simulink model "genericjosephtest"  (Simulink 10.3)
settings: Solver=ode45  StartTime=0.0  StopTime=inf  RelTol=1e-3  EnableMultiTasking=on
values from neighbouring files (symbols this model uses):
  ku = (Lr*m)/(Cyf*(Lf+Lr)) - (Lf*m)/(Cyr*(Lf+Lr))    (= -0.00270204285714)    [makePlants.m]
  Lf = 0.918    [makeBikeModel.m]    (also in makePlants.m)
  Lr = 0.612    [makeBikeModel.m]    (also in makePlants.m)
undefined symbols (not defined in the file or in its folder): Gains
libraries: CarMaker4SL x24, slctrlblks x2, pid_lib x2, simulink x1
(part 2 of 3)

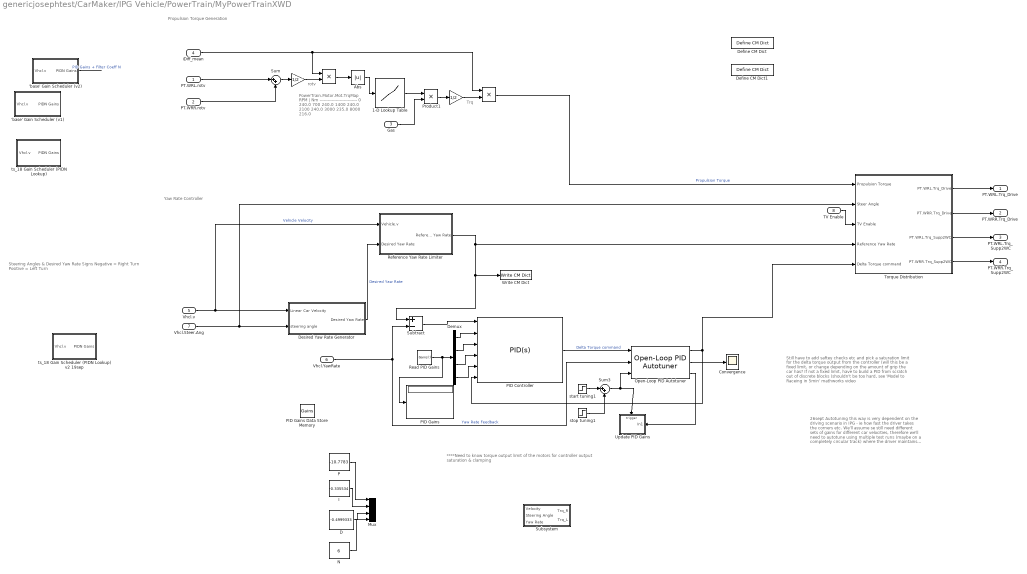
== system genericjosephtest/CarMaker/IPG Vehicle/PowerTrain/MyPowerTrainXWD ==
  note: 26sept
      |
      | Autotuning this way is very dependent on the driving scenario in IPG - ie how fast the driver takes the corners etc. We'll assume se still need different sets of gains for different car velocities, therefore we'll need to autotune using multiple test runs (maybe on a completely circular track) where the driver maintains different cruising speeds each time. Also, need to be mindful of when the start-stop time for the autotuning to ensure the controller is tuned for the correct scenario (ie mid-turn and a relatively constant speed rather than accelerating from a standstill).
      |
      | **also investigate some weird spikes and behaviour of the reference/desired yaw rate generators
  note: Propulsion Torque Generation
  note: ****Need to know torque output limit of the motors for controller output saturation & clamping
  note: Still have to add saftey checks etc and pick a saturation limit for the delta torque output from the controller (will this be a fixed limit, or change depending on the amount of grip the car has? If not a fixed limit, have to build a PID from scratch out of discrete blocks (shouldn't be too hard, see 'Model to Raceing in 5min' mathworks video
  note: Steering Angles & Desired Yaw Rate Signs
      |
      | Negative = Right Turn
      | Positive = Left Turn
  note: rotv
  note: Trq
  note: PowerTrain.Motor.Mot.TrqMap
      |
      |     RPM |  Nm
      | ----------------------------
      |     0         240.0
      |     700     240.0
      |     1400   240.0
      |     2100   240.0
      |     3000   235.0
      |     8000   216.0
  note: Yaw Rate Controller
  PT.WRL.rotv : Inport
  PT.WRR.rotv : Inport  Port=2
  Gas : Inport  Port=3
  iDiff_mean : Inport  Port=4
  Vhcl.v : Inport  Port=5
  Vhcl.YawRate : Inport  Port=6
  Vhcl.Steer.Ang : Inport  Port=7
  TV Enable : Inport  Port=8
  " " : Gain  Gain=1/2
  "  " : Gain  Gain=1/2
  "   " : Product
  "    " : Product
  'base' Gain Scheduler (v1) : Subsystem
  'base' Gain Scheduler (v2) : Subsystem
  1-D Lookup Table : Lookup_n-D  NumberOfTableDimensions=1  BreakpointsForDimension1=[0,700,1400,2100,3000,8000]  Table=[240,240,240,240,235,216]  InternalRulePriority=Speed  RndMeth=Simplest  InputSameDT=on
  Abs : Abs
  Convergence : Scope
  D : Constant  Value=-0.4999333
  Define CM Dict : CarMaker4SL/Define CM Dict  xname=RefYawRate  xunit=rad/s  xmono=off  xtype=Double4  xdvaplace=None  xnstates=0  xfirststate=0  xinitial=0
  Define CM Dict1 : CarMaker4SL/Define CM Dict  xname=DesYawRate  xunit=rad/s  xmono=off  xtype=Double4  xdvaplace=None  xnstates=0  xfirststate=0  xinitial=0
  Demux : Demux
  Desired Yaw Rate Generator : Subsystem
  I : Constant  Value=-0.335534
  Mux : Mux
  N : Constant  Value=6
  Open-Loop PID Autotuner : slctrlblks/Open-Loop PID Autotuner  PIDType=PIDF  PIDForm=Parallel  TimeDomain=discrete-time  DiscreteTs=0.1  IntegratorFormula=Forward Euler  FilterFormula=Forward Euler  ContinuousTs=0.02  Bandwidth=2  UseExternalWC=off  TargetPM=60  UseExternalPM=off  UseExternalAchievedPM=off  AmpSine=0.1  UseExternalAmpSine=off  EstimateDCGain=on  AmpStep=0.1  UseExternalAmpStep=off  UseExternalFRD=off  UseExternalU0=off  UseExternalDCGain=off  NotDeployTuningModule=off  UsePLCCoder=off  BlockDataType=double  UseConnectedPID=on  blockpath=[]  tunedP=0  tunedI=0  tunedD=0  tunedN=100  tunedPM=0  EstimationWindowSize=4
      settings: SourceProductBaseCode=SD
  P : Constant  Value=-10.7783
  "PID Controller " : pid_lib/PID Controller  Controller=PID  Form=Parallel  TimeDomain=Continuous-time  UseExternalTs=off  SampleTime=-1  IntegratorMethod=Forward Euler  FilterMethod=Forward Euler  ControllerParametersSource=external  P=140  I=2312  D=0.85  UseFilter=on  N=47  TunerSelectOption=Transfer Function Based (PID Tuner App)  InitialConditionSource=internal  InitialConditionForIntegrator=0  InitialConditionForFilter=0  DifferentiatorICPrevScaledInput=0  ExternalReset=none  TrackingMode=on  Kt=1  LimitOutput=off  SatLimitsSource=internal  UpperSaturationLimit=240  LowerSaturationLimit=0  LinearizeAsGain=off  AntiWindupMode=clamping  Kb=1  POutMin=[]  POutMax=[]  IOutMin=[]  IOutMax=[]  DOutMin=[]  DOutMax=[]  NOutMin=[]  NOutMax=[]  SumOutMin=[]  SumOutMax=[]  SaturationOutMin=[]  SaturationOutMax=[]  PParamMin=[]  PParamMax=[]  IParamMin=[]  IParamMax=[]  DParamMin=[]  DParamMax=[]  NParamMin=[]  NParamMax=[]  KbParamMin=[]  KbParamMax=[]  KtParamMin=[]  KtParamMax=[]  KbOutMin=[]  KbOutMax=[]  KtOutMin=[]  KtOutMax=[]  IntegratorOutMin=[]  IntegratorOutMax=[]  FilterOutMin=[]  FilterOutMax=[]  SumI1OutMin=[]  SumI1OutMax=[]  SumI2OutMin=[]  SumI2OutMax=[]  SumI3OutMin=[]  SumI3OutMax=[]  SumI4OutMin=[]  SumI4OutMax=[]  SumDOutMin=[]  SumDOutMax=[]  DifferentiatorOutMin=[]  DifferentiatorOutMax=[]  FilterDiffOutCoefMin=[]  FilterDiffOutCoefMax=[]  ReciprocalOutMin=[]  ReciprocalOutMax=[]  SumDenOutMin=[]  SumDenOutMax=[]  SumNumOutMin=[]  SumNumOutMax=[]  DivideOutMin=[]  DivideOutMax=[]  UdiffTsProdOutMin=[]  UdiffTsProdOutMax=[]  NTsProdOutMin=[]  NTsProdOutMax=[]  UintegralTsProdOutMin=[]  UintegralTsProdOutMax=[]  UngainTsProdOutMin=[]  UngainTsProdOutMax=[]  IntegratorContinuousStateAttributes=''  IntegratorStateMustResolveToSignalObject=off  IntegratorRTWStateStorageClass=Auto  FilterContinuousStateAttributes=''  FilterStateMustResolveToSignalObject=off  FilterRTWStateStorageClass=Auto  ParallelPVariant=ExternalParameters  IdealPVariant=Disabled  IVariant=ExternalParameters  DVariant=ExternalParameters  IntegratorVariant=Continuous  SatVariant=Disabled  AWVariant=Passthrough  PCopyVariant=Disabled  TRVariant=Enabled  FdbkBlocksVariant=Forward  IdealPFdbkVariant=Disabled  SatFdbkVariant=Disabled  DerivativeFilterVariant=ContFilter  NVariant=ExternalParameters  NCopyVariant=Disabled  FilterICVariant=InternalICsFilter  IntegratorICVariant=InternalICs  ExternalResetVariant=Disabled  TRSumVariant=TrackingMode  SumFdbkVariant=Disabled  SumVariant=Sum_PID  TsampFilterVariant=InternalTs  TsampNgainVariant=Passthrough  TsampIntegralVariant=Passthrough  ExternalSaturationOutDataTypeStr=Inherit: Same as second input
  PID Gains : Display
      settings: Decimation=5
  PID Gains Data Store Memory : DataStoreMemory  DataStoreName=Gains  InitialValue=[120 120 120 120]  ShowAdditionalParam=off
  Product1 : Product  RndMeth=Zero
  Read PID Gains : DataStoreRead  DataStoreName=Gains  DataStoreElements=Gains(:)  IndexOptions=Index vector (dialog)  Indices=1  OutputSizes=1
  Reference Yaw Rate Limiter : Subsystem
  Subsystem : Subsystem
  Subtract : Sum  Inputs=+-
  Sum : Sum  Inputs=|++
  Sum3 : Sum  Inputs=|++
  Torque Distribution : Subsystem
  Update PID Gains : Subsystem
  Write CM Dict : CarMaker4SL/Write CM Dict  xname=RefYawRate  xsync=off
  start tuning1 : Step  Time=10  SampleTime=0
  stop tuning1 : Step  Time=28  After=-1  SampleTime=0
  ts_18 Gain Scheduler (PIDN Lookup) : Subsystem
  ts_18 Gain Scheduler (PIDN Lookup) v2 19sep : Subsystem
  PT.WRL.Trq_Drive : Outport  VectorParamsAs1DForOutWhenUnconnected=off
  PT.WRR.Trq_Drive : Outport  Port=2  VectorParamsAs1DForOutWhenUnconnected=off
  PT.WRL.Trq_Supp2WC : Outport  Port=3  VectorParamsAs1DForOutWhenUnconnected=off
  PT.WRR.Trq_Supp2WC : Outport  Port=4  VectorParamsAs1DForOutWhenUnconnected=off
  wires:
  "  "/1 -> "   "/2
  Product1/1 -> "  "/1
  Gas/1 -> Product1/2
  1-D Lookup Table/1 -> Product1/1
  "    "/1 -> Abs/1
  iDiff_mean/1 -> "   "/1, "    "/1
  " "/1 -> "    "/2
  Sum/1 -> " "/1
  PT.WRR.rotv/1 -> Sum/2
  PT.WRL.rotv/1 -> Sum/1
  Abs/1 -> 1-D Lookup Table/1
  Vhcl.v/1 -> Desired Yaw Rate Generator/1(Linear Car Velocity), Reference Yaw Rate Limiter/1(Vehicle.v)  "Vehicle Velocity"
  Vhcl.Steer.Ang/1 -> Torque Distribution/2(Steer Angle), Desired Yaw Rate Generator/2(steering angle)
  Desired Yaw Rate Generator/1(Desired Yaw Rate) -> Reference Yaw Rate Limiter/2(Desired Yaw Rate)  "Desired Yaw Rate"
  Vhcl.YawRate/1 -> Open-Loop PID Autotuner/2, Subtract/2  "Yaw Rate Feedback"
  "   "/1 -> Torque Distribution/1(Propulsion Torque)  "Propulsion Torque"
  TV Enable/1 -> Torque Distribution/3(TV Enable)
  Torque Distribution/1(PT.WRL.Trq_Drive) -> PT.WRL.Trq_Drive/1
  Torque Distribution/2(PT.WRR.Trq_Drive) -> PT.WRR.Trq_Drive/1
  Torque Distribution/3(PT.WRL.Trq_Supp2WC) -> PT.WRL.Trq_Supp2WC/1
  Torque Distribution/4(PT.WRR.Trq_Supp2WC) -> PT.WRR.Trq_Supp2WC/1
  Reference Yaw Rate Limiter/1(Reference Yaw Rate) -> Write CM Dict/1, Subtract/1, Torque Distribution/4(Reference Yaw Rate)
  Demux/1 -> "PID Controller "/2
  Demux/2 -> "PID Controller "/3
  Demux/3 -> "PID Controller "/4
  Demux/4 -> "PID Controller "/5
  Subtract/1 -> "PID Controller "/1
  'base' Gain Scheduler (v2)/1(PIDN Gains) -> ?  "PID Gains + Filter Coeff N"
  Read PID Gains/1 -> Demux/1, PID Gains/1
  stop tuning1/1 -> Sum3/2
  start tuning1/1 -> Sum3/1
  Sum3/1 -> Update PID Gains/Trigger, Open-Loop PID Autotuner/3
  Open-Loop PID Autotuner/3 -> Update PID Gains/1(In1)
  Open-Loop PID Autotuner/2 -> Convergence/1
  P/1 -> Mux/1
  I/1 -> Mux/2
  D/1 -> Mux/3
  N/1 -> Mux/4
  "PID Controller "/1 -> Open-Loop PID Autotuner/1  "Delta Torque command"
  Open-Loop PID Autotuner/1 -> Torque Distribution/5(Delta Torque command), "PID Controller "/6

== system genericjosephtest/CarMaker/IPG Vehicle/CarAndTrailer/CarAndTrailerUpd/CreateBus Brake.IF.In ==
  In : Inport
  BusCreator : BusCreator  Inputs=9
  Demux : Demux  Outputs=9
      settings: DisplayOption=none
  Out : Outport  VectorParamsAs1DForOutWhenUnconnected=off
  wires:
  Demux/9 -> BusCreator/9  "Brake IF Trq_Reg RR"
  Demux/8 -> BusCreator/8  "Brake IF Trq_Reg RL"
  Demux/7 -> BusCreator/7  "Brake IF Trq_Reg FR"
  Demux/6 -> BusCreator/6  "Brake IF Trq_Reg FL"
  Demux/5 -> BusCreator/5  "Brake IF Trq_Reg_max RR"
  Demux/4 -> BusCreator/4  "Brake IF Trq_Reg_max RL"
  Demux/3 -> BusCreator/3  "Brake IF Trq_Reg_max FR"
  Demux/2 -> BusCreator/2  "Brake IF Trq_Reg_max FL"
  Demux/1 -> BusCreator/1  "Brake IF T_env"
  BusCreator/1 -> Out/1
  In/1 -> Demux/1

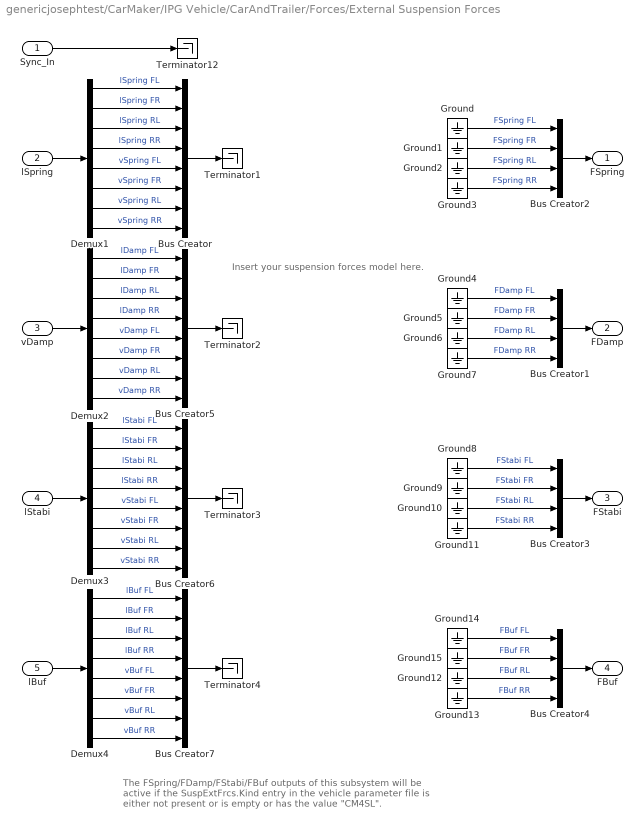
== system genericjosephtest/CarMaker/IPG Vehicle/CarAndTrailer/Forces/External Suspension Forces ==
  note: The FSpring/FDamp/FStabi/FBuf outputs of this subsystem will be
      | active if the SuspExtFrcs.Kind entry in the vehicle parameter file
      | is either not present or is empty or has the value "CM4SL".
  note: Insert your suspension forces model here.
  Sync_In : Inport
  lSpring : Inport  Port=2
  vDamp : Inport  Port=3
  lStabi : Inport  Port=4
  lBuf : Inport  Port=5
  Bus Creator{,5..7} (4 alike) : BusCreator  Inputs=8
  Bus Creator{1..4} (4 alike) : BusCreator  Inputs=4
  Demux{1..4} (4 alike) : Demux  Outputs=8
      settings: DisplayOption=none
  Ground{,1..15} (16 alike) : Ground
  Terminator{1..4,12} (5 alike) : Terminator
  FSpring : Outport  VectorParamsAs1DForOutWhenUnconnected=off
  FDamp : Outport  Port=2  VectorParamsAs1DForOutWhenUnconnected=off
  FStabi : Outport  Port=3  VectorParamsAs1DForOutWhenUnconnected=off
  FBuf : Outport  Port=4  VectorParamsAs1DForOutWhenUnconnected=off
  wires:
  Bus Creator7/1 -> Terminator4/1
  Bus Creator6/1 -> Terminator3/1
  Bus Creator5/1 -> Terminator2/1
  Bus Creator/1 -> Terminator1/1
  Demux4/8 -> Bus Creator7/8  "vBuf RR"
  Demux4/7 -> Bus Creator7/7  "vBuf RL"
  Demux4/6 -> Bus Creator7/6  "vBuf FR"
  Demux4/5 -> Bus Creator7/5  "vBuf FL"
  Demux3/8 -> Bus Creator6/8  "vStabi RR"
  Demux3/7 -> Bus Creator6/7  "vStabi RL"
  Demux3/6 -> Bus Creator6/6  "vStabi FR"
  Demux3/5 -> Bus Creator6/5  "vStabi FL"
  Demux2/8 -> Bus Creator5/8  "vDamp RR"
  Demux2/7 -> Bus Creator5/7  "vDamp RL"
  Demux2/6 -> Bus Creator5/6  "vDamp FR"
  Demux2/5 -> Bus Creator5/5  "vDamp FL"
  Demux1/8 -> Bus Creator/8  "vSpring RR"
  Demux1/7 -> Bus Creator/7  "vSpring RL"
  Demux1/6 -> Bus Creator/6  "vSpring FR"
  Demux1/5 -> Bus Creator/5  "vSpring FL"
  Demux2/4 -> Bus Creator5/4  "lDamp RR"
  Demux2/3 -> Bus Creator5/3  "lDamp RL"
  Demux2/2 -> Bus Creator5/2  "lDamp FR"
  Demux2/1 -> Bus Creator5/1  "lDamp FL"
  Demux1/4 -> Bus Creator/4  "lSpring RR"
  Demux1/3 -> Bus Creator/3  "lSpring RL"
  Demux1/2 -> Bus Creator/2  "lSpring FR"
  Demux1/1 -> Bus Creator/1  "lSpring FL"
  Demux3/4 -> Bus Creator6/4  "lStabi RR"
  Demux3/3 -> Bus Creator6/3  "lStabi RL"
  Demux3/2 -> Bus Creator6/2  "lStabi FR"
  Demux3/1 -> Bus Creator6/1  "lStabi FL"
  lStabi/1 -> Demux3/1
  vDamp/1 -> Demux2/1
  lSpring/1 -> Demux1/1
  Demux4/4 -> Bus Creator7/4  "lBuf RR"
  Demux4/3 -> Bus Creator7/3  "lBuf RL"
  Demux4/2 -> Bus Creator7/2  "lBuf FR"
  Demux4/1 -> Bus Creator7/1  "lBuf FL"
  lBuf/1 -> Demux4/1
  Ground14/1 -> Bus Creator4/1  "FBuf FL"
  Ground15/1 -> Bus Creator4/2  "FBuf FR"
  Ground12/1 -> Bus Creator4/3  "FBuf RL"
  Ground13/1 -> Bus Creator4/4  "FBuf RR"
  Bus Creator4/1 -> FBuf/1
  Sync_In/1 -> Terminator12/1
  Bus Creator2/1 -> FSpring/1
  Ground/1 -> Bus Creator2/1  "FSpring FL"
  Ground1/1 -> Bus Creator2/2  "FSpring FR"
  Ground2/1 -> Bus Creator2/3  "FSpring RL"
  Ground3/1 -> Bus Creator2/4  "FSpring RR"
  Ground4/1 -> Bus Creator1/1  "FDamp FL"
  Ground5/1 -> Bus Creator1/2  "FDamp FR"
  Ground6/1 -> Bus Creator1/3  "FDamp RL"
  Ground7/1 -> Bus Creator1/4  "FDamp RR"
  Bus Creator1/1 -> FDamp/1
  Ground8/1 -> Bus Creator3/1  "FStabi FL"
  Ground9/1 -> Bus Creator3/2  "FStabi FR"
  Ground10/1 -> Bus Creator3/3  "FStabi RL"
  Ground11/1 -> Bus Creator3/4  "FStabi RR"
  Bus Creator3/1 -> FStabi/1

== system genericjosephtest/CarMaker/IPG Vehicle/CarAndTrailer/Forces/Tires ==
  note: The TireXX_Out signals will only be used if FileIdent is "CarMaker-Tire-CM4SL" in the tire parameter file!
      | An example parameter file can be found in Data/Tire/DT_CM4SL_UserTire.
  Sync_In : Inport
  TireFL_In : Inport  Port=2
  TireFR_In : Inport  Port=3
  TireRL_In : Inport  Port=4
  TireRR_In : Inport  Port=5
  Bus Creator{1..4} (4 alike) : BusCreator  Inputs=11
  Demux{1..3,8} (4 alike) : Demux  Outputs=7
      settings: DisplayOption=none
  TireFL : Subsystem
  TireFR : Subsystem
  TireRL : Subsystem
  TireRR : Subsystem
  TireFL_Out : Outport  VectorParamsAs1DForOutWhenUnconnected=off
  TireFR_Out : Outport  Port=2  VectorParamsAs1DForOutWhenUnconnected=off
  TireRL_Out : Outport  Port=3  VectorParamsAs1DForOutWhenUnconnected=off
  TireRR_Out : Outport  Port=4  VectorParamsAs1DForOutWhenUnconnected=off
  wires:
  Sync_In/1 -> TireRR/1(Sync_In), TireRL/1(Sync_In), TireFR/1(Sync_In), TireFL/1(Sync_In)
  Bus Creator4/1 -> TireRR_Out/1
  Bus Creator2/1 -> TireRL_Out/1
  Bus Creator1/1 -> TireFR_Out/1
  Demux3/5 -> TireRR/6(Rim_turnv)  "Tire_In Rim_turnv"
  Demux3/4 -> TireRR/5(Rim_rotv)  "Tire_In Rim_rotv"
  Demux3/1 -> TireRR/2(Load)  "Tire_In Load"
  Demux3/7 -> TireRR/8(muRoad)  "Tire_In mu"
  Demux3/6 -> TireRR/7(InclinAngle)  "Tire_In Camber"
  Demux3/2 -> TireRR/3(vxtrans)  "Tire_In vxtrans"
  Demux3/3 -> TireRR/4(vytrans)  "Tire_In vytrans"
  TireRR/11(AlignTrq) -> Bus Creator4/11  "Tire_Out AlignTrq"
  TireRR/10(RollResist) -> Bus Creator4/10  "Tire_Out RollResist"
  TireRR/9(OverturnTrq) -> Bus Creator4/9  "Tire_Out OverturnTrq"
  TireRR/8(LoadFrc) -> Bus Creator4/8  "Tire_Out LoadFrc"
  TireRR/7(SideFrc) -> Bus Creator4/7  "Tire_Out SideFrc"
  TireRR/6(LongFrc) -> Bus Creator4/6  "Tire_Out LongFrc"
  TireRR/5(vBelt) -> Bus Creator4/5  "Tire_Out vBelt"
  TireRR/4(rBelt_eff) -> Bus Creator4/4  "Tire_Out rBelt_eff"
  TireRR/3(TurnSlp) -> Bus Creator4/3  "Tire_Out TurnSlp"
  TireRR/1(Slp) -> Bus Creator4/1  "Tire_Out Slp"
  TireRR/2(Alpha) -> Bus Creator4/2  "Tire_Out Alpha"
  Demux2/5 -> TireRL/6(Rim_turnv)  "Tire_In Rim_turnv"
  Demux2/4 -> TireRL/5(Rim_rotv)  "Tire_In Rim_rotv"
  Demux2/1 -> TireRL/2(Load)  "Tire_In Load"
  Demux2/7 -> TireRL/8(muRoad)  "Tire_In mu"
  Demux2/6 -> TireRL/7(InclinAngle)  "Tire_In Camber"
  Demux2/2 -> TireRL/3(vxtrans)  "Tire_In vxtrans"
  Demux2/3 -> TireRL/4(vytrans)  "Tire_In vytrans"
  TireRL/11(AlignTrq) -> Bus Creator2/11  "Tire_Out AlignTrq"
  TireRL/10(RollResist) -> Bus Creator2/10  "Tire_Out RollResist"
  TireRL/9(OverturnTrq) -> Bus Creator2/9  "Tire_Out OverturnTrq"
  TireRL/8(LoadFrc) -> Bus Creator2/8  "Tire_Out LoadFrc"
  TireRL/7(SideFrc) -> Bus Creator2/7  "Tire_Out SideFrc"
  TireRL/6(LongFrc) -> Bus Creator2/6  "Tire_Out LongFrc"
  TireRL/5(vBelt) -> Bus Creator2/5  "Tire_Out vBelt"
  TireRL/4(rBelt_eff) -> Bus Creator2/4  "Tire_Out rBelt_eff"
  TireRL/3(TurnSlp) -> Bus Creator2/3  "Tire_Out TurnSlp"
  TireRL/1(Slp) -> Bus Creator2/1  "Tire_Out Slp"
  TireRL/2(Alpha) -> Bus Creator2/2  "Tire_Out Alpha"
  Demux1/5 -> TireFR/6(Rim_turnv)  "Tire_In Rim_turnv"
  Demux1/4 -> TireFR/5(Rim_rotv)  "Tire_In Rim_rotv"
  Demux1/1 -> TireFR/2(Load)  "Tire_In Load"
  Demux1/7 -> TireFR/8(muRoad)  "Tire_In mu"
  Demux1/6 -> TireFR/7(InclinAngle)  "Tire_In Camber"
  Demux1/2 -> TireFR/3(vxtrans)  "Tire_In vxtrans"
  Demux1/3 -> TireFR/4(vytrans)  "Tire_In vytrans"
  TireFR/11(AlignTrq) -> Bus Creator1/11  "Tire_Out AlignTrq"
  TireFR/10(RollResist) -> Bus Creator1/10  "Tire_Out RollResist"
  TireFR/9(OverturnTrq) -> Bus Creator1/9  "Tire_Out OverturnTrq"
  TireFR/8(LoadFrc) -> Bus Creator1/8  "Tire_Out LoadFrc"
  TireFR/7(SideFrc) -> Bus Creator1/7  "Tire_Out SideFrc"
  TireFR/6(LongFrc) -> Bus Creator1/6  "Tire_Out LongFrc"
  TireFR/5(vBelt) -> Bus Creator1/5  "Tire_Out vBelt"
  TireFR/4(rBelt_eff) -> Bus Creator1/4  "Tire_Out rBelt_eff"
  TireFR/3(TurnSlp) -> Bus Creator1/3  "Tire_Out TurnSlp"
  TireFR/1(Slp) -> Bus Creator1/1  "Tire_Out Slp"
  TireFR/2(Alpha) -> Bus Creator1/2  "Tire_Out Alpha"
  Demux8/5 -> TireFL/6(Rim_turnv)  "Tire_In Rim_turnv"
  Demux8/4 -> TireFL/5(Rim_rotv)  "Tire_In Rim_rotv"
  TireFL_In/1 -> Demux8/1
  Demux8/1 -> TireFL/2(Load)  "Tire_In Load"
  Demux8/7 -> TireFL/8(muRoad)  "Tire_In mu"
  Demux8/6 -> TireFL/7(InclinAngle)  "Tire_In Camber"
  Demux8/2 -> TireFL/3(vxtrans)  "Tire_In vxtrans"
  Demux8/3 -> TireFL/4(vytrans)  "Tire_In vytrans"
  TireFL/11(AlignTrq) -> Bus Creator3/11  "Tire_Out AlignTrq"
  TireFL/10(RollResist) -> Bus Creator3/10  "Tire_Out RollResist"
  TireFL/9(OverturnTrq) -> Bus Creator3/9  "Tire_Out OverturnTrq"
  TireFL/8(LoadFrc) -> Bus Creator3/8  "Tire_Out LoadFrc"
  TireFL/7(SideFrc) -> Bus Creator3/7  "Tire_Out SideFrc"
  TireFL/6(LongFrc) -> Bus Creator3/6  "Tire_Out LongFrc"
  TireFL/5(vBelt) -> Bus Creator3/5  "Tire_Out vBelt"
  TireFL/4(rBelt_eff) -> Bus Creator3/4  "Tire_Out rBelt_eff"
  TireFL/3(TurnSlp) -> Bus Creator3/3  "Tire_Out TurnSlp"
  TireFL/1(Slp) -> Bus Creator3/1  "Tire_Out Slp"
  TireFL/2(Alpha) -> Bus Creator3/2  "Tire_Out Alpha"
  Bus Creator3/1 -> TireFL_Out/1
  TireFR_In/1 -> Demux1/1
  TireRL_In/1 -> Demux2/1
  TireRR_In/1 -> Demux3/1

== system genericjosephtest/CarMaker/IPG Vehicle/CarAndTrailer/Forces/Vehicle Forces ==
  Sync_In : Inport
  Bus Creator1 : BusCreator  Inputs=12
  Bus Creator8 : BusCreator  Inputs=16
  BusCreator1 : BusCreator  Inputs=4
  BusCreator2 : BusCreator  Inputs=9
  Demux : Demux  Outputs=16
      settings: DisplayOption=none
  Demux1 : Demux  Outputs=12
      settings: DisplayOption=none
  Demux2 : Demux  Outputs=13
      settings: DisplayOption=none
  Forces : S-Function  FunctionName=CM_Sfun  Parameters='Forces'  SFunctionDeploymentMode=off  EnableBusSupport=off
  Terminator : Terminator
  Sync_Out : Outport  VectorParamsAs1DForOutWhenUnconnected=off
  Car.Virtual : Outport  Port=2  VectorParamsAs1DForOutWhenUnconnected=off
  Car.Aero : Outport  Port=3  VectorParamsAs1DForOutWhenUnconnected=off
  Car.Load : Outport  Port=4  VectorParamsAs1DForOutWhenUnconnected=off
  wires:
  BusCreator1/1 -> Terminator/1  "Aero IF (in)"
  Demux2/13 -> BusCreator2/9  "car Aero Trq_1 z"
  Demux2/12 -> BusCreator2/8  "car Aero Trq_1 y"
  Demux2/11 -> BusCreator2/7  "car Aero Trq_1 x"
  Demux2/10 -> BusCreator2/6  "car Aero Frc_1 z"
  Demux2/9 -> BusCreator2/5  "car Aero Frc_1 y"
  Demux2/8 -> BusCreator2/4  "car Aero Frc_1 x"
  Demux2/7 -> BusCreator2/3  "car Aero PoA_1 z"
  Demux2/6 -> BusCreator2/2  "car Aero PoA_1 y"
  Demux2/5 -> BusCreator2/1  "car Aero PoA_1 x"
  Demux2/4 -> BusCreator1/4  "car Aero tau_1"
  Demux2/3 -> BusCreator1/3  "car Aero ApproachVel_1 z"
  Demux2/2 -> BusCreator1/2  "car Aero ApproachVel_1 y"
  Demux2/1 -> BusCreator1/1  "car Aero ApproachVel_1 x"
  Demux/16 -> Bus Creator8/16  "Car Load_3 tz"
  Demux/15 -> Bus Creator8/15  "Car Load_3 ty"
  Demux/14 -> Bus Creator8/14  "Car Load_3 tx"
  Demux/13 -> Bus Creator8/13  "Car Load_3 mass"
  Demux1/12 -> Bus Creator1/12  "Car Virtual Trq_0 z"
  Demux1/11 -> Bus Creator1/11  "Car Virtual Trq_0 y"
  Demux1/10 -> Bus Creator1/10  "Car Virtual Trq_0 x"
  Demux1/9 -> Bus Creator1/9  "Car Virtual Trq_1 z"
  Demux1/8 -> Bus Creator1/8  "Car Virtual Trq_1 y"
  Demux1/7 -> Bus Creator1/7  "Car Virtual Trq_1 x"
  Demux1/6 -> Bus Creator1/6  "Car Virtual Frc_0 z"
  Demux1/5 -> Bus Creator1/5  "Car Virtual Frc_0 y"
  Demux1/4 -> Bus Creator1/4  "Car Virtual Frc_0 x"
  Sync_In/1 -> Forces/1
  Forces/1 -> Sync_Out/1
  BusCreator2/1 -> Car.Aero/1
  Demux1/1 -> Bus Creator1/1  "Car Virtual Frc_1 x"
  Demux1/2 -> Bus Creator1/2  "Car Virtual Frc_1 y"
  Demux1/3 -> Bus Creator1/3  "Car Virtual Frc_1 z"
  Forces/3 -> Demux2/1
  Forces/2 -> Demux1/1
  Bus Creator1/1 -> Car.Virtual/1
  Bus Creator8/1 -> Car.Load/1
  Demux/1 -> Bus Creator8/1  "Car Load_0 mass"
  Demux/2 -> Bus Creator8/2  "Car Load_0 tx"
  Demux/3 -> Bus Creator8/3  "Car Load_0 ty"
  Demux/4 -> Bus Creator8/4  "Car Load_0 tz"
  Demux/5 -> Bus Creator8/5  "Car Load_1 mass"
  Demux/6 -> Bus Creator8/6  "Car Load_1 tx"
  Demux/7 -> Bus Creator8/7  "Car Load_1 ty"
  Demux/8 -> Bus Creator8/8  "Car Load_1 tz"
  Demux/9 -> Bus Creator8/9  "Car Load_2 mass"
  Demux/10 -> Bus Creator8/10  "Car Load_2 tx"
  Demux/11 -> Bus Creator8/11  "Car Load_2 ty"
  Demux/12 -> Bus Creator8/12  "Car Load_2 tz"
  Forces/4 -> Demux/1

== system genericjosephtest/CarMaker/IPG Vehicle/CarAndTrailer/Trailer/CreateBus Car.Hitch.FrcTrq ==
  In1 : Inport
  Bus Creator7 : BusCreator  Inputs=6
  Demux7 : Demux  Outputs=6
      settings: DisplayOption=none
  Out1 : Outport  VectorParamsAs1DForOutWhenUnconnected=off
  wires:
  In1/1 -> Demux7/1
  Bus Creator7/1 -> Out1/1
  Demux7/6 -> Bus Creator7/6  "Car Hitch Trq2Car z"
  Demux7/5 -> Bus Creator7/5  "Car Hitch Trq2Car y"
  Demux7/4 -> Bus Creator7/4  "Car Hitch Trq2Car x"
  Demux7/3 -> Bus Creator7/3  "Car Hitch Frc2Car z"
  Demux7/2 -> Bus Creator7/2  "Car Hitch Frc2Car y"
  Demux7/1 -> Bus Creator7/1  "Car Hitch Frc2Car x"

== system genericjosephtest/CarMaker/IPG Vehicle/CarAndTrailer/Trailer/CreateBus Vhcl.Motion ==
  In1 : Inport
  BusCreator : BusCreator  Inputs=15
  Demux : Demux  Outputs=15
      settings: DisplayOption=none
  Out1 : Outport  VectorParamsAs1DForOutWhenUnconnected=off
  wires:
  Demux/15 -> BusCreator/15  "Vhcl YawAcc"
  Demux/14 -> BusCreator/14  "Vhcl YawVel"
  Demux/13 -> BusCreator/13  "Vhcl Yaw"
  Demux/12 -> BusCreator/12  "Vhcl PitchAcc"
  Demux/11 -> BusCreator/11  "Vhcl PitchVel"
  Demux/10 -> BusCreator/10  "Vhcl Pitch"
  Demux/9 -> BusCreator/9  "Vhcl RollAcc"
  Demux/8 -> BusCreator/8  "Vhcl RollVel"
  Demux/7 -> BusCreator/7  "Vhcl Roll"
  Demux/6 -> BusCreator/6  "Vhcl Hitch_Pos z"
  Demux/5 -> BusCreator/5  "Vhcl Hitch_Pos y"
  Demux/4 -> BusCreator/4  "Vhcl Hitch_Pos x"
  Demux/3 -> BusCreator/3  "Vhcl sRoad"
  Demux/2 -> BusCreator/2  "Vhcl Distance"
  Demux/1 -> BusCreator/1  "Vhcl v"
  In1/1 -> Demux/1
  BusCreator/1 -> Out1/1

== system genericjosephtest/CarMaker/IPG Vehicle/CarAndTrailer/Trailer/CreateBus Vhcl.PoI ==
  In1 : Inport
  Bus Creator3 : BusCreator  Inputs=18
  Demux3 : Demux  Outputs=18
      settings: DisplayOption=none
  Out1 : Outport  VectorParamsAs1DForOutWhenUnconnected=off
  wires:
  Demux3/18 -> Bus Creator3/18  "Vhcl PoI_GCS Elev"
  Demux3/17 -> Bus Creator3/17  "Vhcl PoI_GCS Lat"
  Demux3/16 -> Bus Creator3/16  "Vhcl PoI_GCS Long"
  Demux3/15 -> Bus Creator3/15  "Vhcl PoI_Acc_1 z"
  Demux3/14 -> Bus Creator3/14  "Vhcl PoI_Acc_1 y"
  Demux3/13 -> Bus Creator3/13  "Vhcl PoI_Acc_1 x"
  Demux3/12 -> Bus Creator3/12  "Vhcl PoI_Vel_1 z"
  Demux3/11 -> Bus Creator3/11  "Vhcl PoI_Vel_1 y"
  Demux3/10 -> Bus Creator3/10  "Vhcl PoI_Vel_1 x"
  Demux3/9 -> Bus Creator3/9  "Vhcl PoI_Acc z"
  Demux3/8 -> Bus Creator3/8  "Vhcl PoI_Acc y"
  Demux3/7 -> Bus Creator3/7  "Vhcl PoI_Acc x"
  Demux3/6 -> Bus Creator3/6  "Vhcl PoI_Vel z"
  Demux3/5 -> Bus Creator3/5  "Vhcl PoI_Vel y"
  Demux3/4 -> Bus Creator3/4  "Vhcl PoI_Vel x"
  Demux3/3 -> Bus Creator3/3  "Vhcl PoI_Pos z"
  Demux3/2 -> Bus Creator3/2  "Vhcl PoI_Pos y"
  In1/1 -> Demux3/1
  Bus Creator3/1 -> Out1/1
  Demux3/1 -> Bus Creator3/1  "Vhcl PoI_Pos x"

== system genericjosephtest/CarMaker/IPG Vehicle/CarAndTrailer/Trailer/CreateBus Vhcl.Steering ==
  In1 : Inport
  Bus Creator3 : BusCreator  Inputs=4
  Demux : Demux
      settings: DisplayOption=none
  Out1 : Outport  VectorParamsAs1DForOutWhenUnconnected=off
  wires:
  Bus Creator3/1 -> Out1/1
  Demux/1 -> Bus Creator3/1  "Vhcl Steering Ang"
  Demux/3 -> Bus Creator3/3  "Vhcl Steering AngAcc"
  Demux/2 -> Bus Creator3/2  "Vhcl Steering AngVel"
  Demux/4 -> Bus Creator3/4  "Vhcl Steering Trq"
  In1/1 -> Demux/1

== system genericjosephtest/CarMaker/IPG Vehicle/CarAndTrailer/Trailer/CreateBus Vhcl.Wheel.FL ==
  In1 : Inport
  Bus Creator3 : BusCreator  Inputs=14
  Demux3 : Demux  Outputs=14
      settings: DisplayOption=none
  Out1 : Outport  VectorParamsAs1DForOutWhenUnconnected=off
  wires:
  Demux3/14 -> Bus Creator3/14  "Vhcl Wheel FL Trq_WhlBearing"
  Demux3/13 -> Bus Creator3/13  "Vhcl Wheel FL Trq_T2W"
  Demux3/12 -> Bus Creator3/12  "Vhcl Wheel FL SideSlip"
  Demux3/11 -> Bus Creator3/11  "Vhcl Wheel FL LongSlip"
  Demux3/10 -> Bus Creator3/10  "Vhcl Wheel FL vBelt"
  Demux3/9 -> Bus Creator3/9  "Vhcl Wheel FL Fz"
  Demux3/8 -> Bus Creator3/8  "Vhcl Wheel FL Fy"
  Demux3/7 -> Bus Creator3/7  "Vhcl Wheel FL Fx"
  Demux3/6 -> Bus Creator3/6  "Vhcl Wheel FL r_zxy z"
  Demux3/5 -> Bus Creator3/5  "Vhcl Wheel FL r_zxy y"
  Demux3/4 -> Bus Creator3/4  "Vhcl Wheel FL r_zxy x"
  Demux3/3 -> Bus Creator3/3  "Vhcl Wheel FL t z"
  Demux3/2 -> Bus Creator3/2  "Vhcl Wheel FL t y"
  In1/1 -> Demux3/1
  Bus Creator3/1 -> Out1/1
  Demux3/1 -> Bus Creator3/1  "Vhcl Wheel FL t x"

== system genericjosephtest/CarMaker/IPG Vehicle/CarAndTrailer/Trailer/CreateBus Vhcl.Wheel.FR ==
  In1 : Inport
  Bus Creator3 : BusCreator  Inputs=14
  Demux3 : Demux  Outputs=14
      settings: DisplayOption=none
  Out1 : Outport  VectorParamsAs1DForOutWhenUnconnected=off
  wires:
  Demux3/14 -> Bus Creator3/14  "Vhcl Wheel FR Trq_WhlBearing"
  Demux3/13 -> Bus Creator3/13  "Vhcl Wheel FR Trq_T2W"
  Demux3/12 -> Bus Creator3/12  "Vhcl Wheel FR SideSlip"
  Demux3/11 -> Bus Creator3/11  "Vhcl Wheel FR LongSlip"
  Demux3/10 -> Bus Creator3/10  "Vhcl Wheel FR vBelt"
  Demux3/9 -> Bus Creator3/9  "Vhcl Wheel FR Fz"
  Demux3/8 -> Bus Creator3/8  "Vhcl Wheel FR Fy"
  Demux3/7 -> Bus Creator3/7  "Vhcl Wheel FR Fx"
  Demux3/6 -> Bus Creator3/6  "Vhcl Wheel FR r_zxy z"
  Demux3/5 -> Bus Creator3/5  "Vhcl Wheel FR r_zxy y"
  Demux3/4 -> Bus Creator3/4  "Vhcl Wheel FR r_zxy x"
  Demux3/3 -> Bus Creator3/3  "Vhcl Wheel FR t z"
  Demux3/2 -> Bus Creator3/2  "Vhcl Wheel FR t y"
  In1/1 -> Demux3/1
  Bus Creator3/1 -> Out1/1
  Demux3/1 -> Bus Creator3/1  "Vhcl Wheel FR t x"

== system genericjosephtest/CarMaker/IPG Vehicle/CarAndTrailer/Trailer/CreateBus Vhcl.Wheel.RL ==
  In1 : Inport
  Bus Creator3 : BusCreator  Inputs=14
  Demux3 : Demux  Outputs=14
      settings: DisplayOption=none
  Out1 : Outport  VectorParamsAs1DForOutWhenUnconnected=off
  wires:
  Demux3/14 -> Bus Creator3/14  "Vhcl Wheel RL Trq_WhlBearing"
  Demux3/13 -> Bus Creator3/13  "Vhcl Wheel RL Trq_T2W"
  Demux3/12 -> Bus Creator3/12  "Vhcl Wheel RL SideSlip"
  Demux3/11 -> Bus Creator3/11  "Vhcl Wheel RL LongSlip"
  Demux3/10 -> Bus Creator3/10  "Vhcl Wheel RL vBelt"
  Demux3/9 -> Bus Creator3/9  "Vhcl Wheel RL Fz"
  Demux3/8 -> Bus Creator3/8  "Vhcl Wheel RL Fy"
  Demux3/7 -> Bus Creator3/7  "Vhcl Wheel RL Fx"
  Demux3/6 -> Bus Creator3/6  "Vhcl Wheel RL r_zxy z"
  Demux3/5 -> Bus Creator3/5  "Vhcl Wheel RL r_zxy y"
  Demux3/4 -> Bus Creator3/4  "Vhcl Wheel RL r_zxy x"
  Demux3/3 -> Bus Creator3/3  "Vhcl Wheel RL t z"
  Demux3/2 -> Bus Creator3/2  "Vhcl Wheel RL t y"
  In1/1 -> Demux3/1
  Bus Creator3/1 -> Out1/1
  Demux3/1 -> Bus Creator3/1  "Vhcl Wheel RL t x"

== system genericjosephtest/CarMaker/IPG Vehicle/CarAndTrailer/Trailer/CreateBus Vhcl.Wheel.RR ==
  In1 : Inport
  Bus Creator3 : BusCreator  Inputs=14
  Demux3 : Demux  Outputs=14
      settings: DisplayOption=none
  Out1 : Outport  VectorParamsAs1DForOutWhenUnconnected=off
  wires:
  Demux3/14 -> Bus Creator3/14  "Vhcl Wheel RR Trq_WhlBearing"
  Demux3/13 -> Bus Creator3/13  "Vhcl Wheel RR Trq_T2W"
  Demux3/12 -> Bus Creator3/12  "Vhcl Wheel RR SideSlip"
  Demux3/11 -> Bus Creator3/11  "Vhcl Wheel RR LongSlip"
  Demux3/10 -> Bus Creator3/10  "Vhcl Wheel RR vBelt"
  Demux3/9 -> Bus Creator3/9  "Vhcl Wheel RR Fz"
  Demux3/8 -> Bus Creator3/8  "Vhcl Wheel RR Fy"
  Demux3/7 -> Bus Creator3/7  "Vhcl Wheel RR Fx"
  Demux3/6 -> Bus Creator3/6  "Vhcl Wheel RR r_zxy z"
  Demux3/5 -> Bus Creator3/5  "Vhcl Wheel RR r_zxy y"
  Demux3/4 -> Bus Creator3/4  "Vhcl Wheel RR r_zxy x"
  Demux3/3 -> Bus Creator3/3  "Vhcl Wheel RR t z"
  Demux3/2 -> Bus Creator3/2  "Vhcl Wheel RR t y"
  In1/1 -> Demux3/1
  Bus Creator3/1 -> Out1/1
  Demux3/1 -> Bus Creator3/1  "Vhcl Wheel RR t x"

== system genericjosephtest/CarMaker/IPG Vehicle/PowerTrain/MyPowerTrainXWD/'base' Gain Scheduler (v1) ==
  Vhcl.v : Inport
  Kd Lookup : Lookup_n-D  NumberOfTableDimensions=1  BreakpointsForDimension1=[1,3,5,7,9,11,13,15]  Table=[0,0,-7.97,-5.4677,-0.031525,-11.8165,-3.65,-0.34472]  InternalRulePriority=Speed  RndMeth=Simplest  InputSameDT=on
  Ki Lookup : Lookup_n-D  NumberOfTableDimensions=1  BreakpointsForDimension1=[1,3,5,7,9,11,13,15]  Table=[113386.3639,53139.3625,39431.5219,38685.5046,41858.1647,35177.4525,42819.4908,44127.9844]  InternalRulePriority=Speed  RndMeth=Simplest  InputSameDT=on
  Kp Lookup : Lookup_n-D  NumberOfTableDimensions=1  BreakpointsForDimension1=[1,3,5,7,9,11,13,15]  Table=[0,201.9987,715,1006.2519,1334.3392,1559.4809,1823.2205,1917.1532]  InternalRulePriority=Speed  RndMeth=Simplest  InputSameDT=on
  Mux : Mux
  N Lookup : Lookup_n-D  NumberOfTableDimensions=1  BreakpointsForDimension1=[1,3,5,7,9,11,13,15]  Table=[100,100,25.9478,36.7197,4232.6962,38.2401,499.5103,5561.304]  InternalRulePriority=Speed  RndMeth=Simplest  InputSameDT=on
  PIDN Gains : Outport  VectorParamsAs1DForOutWhenUnconnected=off
  wires:
  Vhcl.v/1 -> N Lookup/1, Kd Lookup/1, Ki Lookup/1, Kp Lookup/1
  N Lookup/1 -> Mux/4
  Ki Lookup/1 -> Mux/2
  Kp Lookup/1 -> Mux/1
  Kd Lookup/1 -> Mux/3
  Mux/1 -> PIDN Gains/1

== system genericjosephtest/CarMaker/IPG Vehicle/PowerTrain/MyPowerTrainXWD/'base' Gain Scheduler (v2) ==
  Vhcl.v : Inport
  Kd Lookup : Lookup_n-D  NumberOfTableDimensions=1  BreakpointsForDimension1=[1,3,5,7,9,11,13,15]  Table=[0,0,0,0,0,0,0,0]  InterpMethod=Nearest  InternalRulePriority=Speed  RndMeth=Simplest  InputSameDT=on
  Ki Lookup : Lookup_n-D  NumberOfTableDimensions=1  BreakpointsForDimension1=[1,3,5,7,9,11,13,15]  Table=[575414.9239,182260.6677,104061.59,70206.68,51512.3181,39932.8377,32134.3505,38079.8684]  InterpMethod=Nearest  InternalRulePriority=Speed  RndMeth=Simplest  InputSameDT=on
  Kp Lookup : Lookup_n-D  NumberOfTableDimensions=1  BreakpointsForDimension1=[1,3,5,7,9,11,13,15]  Table=[0,0,2000,2000,0,0,0,0]  InterpMethod=Nearest  InternalRulePriority=Speed  RndMeth=Simplest  InputSameDT=on
  Mux : Mux
  N Lookup : Lookup_n-D  NumberOfTableDimensions=1  BreakpointsForDimension1=[1,3,5,7,9,11,13,15]  Table=[100,100,100,100,100,100,100,100]  InterpMethod=Nearest  InternalRulePriority=Speed  RndMeth=Simplest  InputSameDT=on
  PIDN Gains : Outport  VectorParamsAs1DForOutWhenUnconnected=off
  wires:
  Vhcl.v/1 -> N Lookup/1, Kd Lookup/1, Ki Lookup/1, Kp Lookup/1
  N Lookup/1 -> Mux/4
  Ki Lookup/1 -> Mux/2
  Kp Lookup/1 -> Mux/1
  Kd Lookup/1 -> Mux/3
  Mux/1 -> PIDN Gains/1

== system genericjosephtest/CarMaker/IPG Vehicle/PowerTrain/MyPowerTrainXWD/Desired Yaw Rate Generator ==
  Linear Car Velocity : Inport
  steering angle : Inport  Port=2
  Add : Sum  Inputs=+++
  Constant : Constant  Value=Lf
  Constant1 : Constant  Value=ku
  Constant2 : Constant  Value=Lr
  Define CM Dict : CarMaker4SL/Define CM Dict  xname=desYaw_denom  xmono=off  xtype=Double4  xdvaplace=None  xnstates=0  xfirststate=0  xinitial=0
  Define CM Dict1 : CarMaker4SL/Define CM Dict  xname=desYaw_num  xmono=off  xtype=Double4  xdvaplace=None  xnstates=0  xfirststate=0  xinitial=0
  Divide : Product  Inputs=*/
  Multiply : Product
  Multiply1 : Product
  Square : Math  Operator=square  SignedPower=on  SaturateOnIntegerOverflow=on
  Desired Yaw Rate : Outport  VectorParamsAs1DForOutWhenUnconnected=off
  wires:
  Constant1/1 -> Multiply/1
  steering angle/1 -> Multiply1/2
  Divide/1 -> Desired Yaw Rate/1
  Linear Car Velocity/1 -> Square/1, Multiply1/1
  Multiply/1 -> Add/1
  Multiply1/1 -> Divide/1
  Square/1 -> Multiply/2
  Constant/1 -> Add/2
  Constant2/1 -> Add/3
  Add/1 -> Divide/2

== system genericjosephtest/CarMaker/IPG Vehicle/PowerTrain/MyPowerTrainXWD/Reference Yaw Rate Limiter ==
  note: Bind the reference yaw rate to the max possible yaw rate if the desired yaw rate is more than the max yaw rate possible
  note: Max Yaw Rate = tunability*mu*g/Vcg
  Vehicle.v : Inport
  Desired Yaw Rate : Inport  Port=2
  Add : Sum
  Constant : Constant  Value=2
  Constant1 : Constant  Value=0
  Define CM Dict : CarMaker4SL/Define CM Dict  xname=maxYawRate  xmono=off  xtype=Double4  xdvaplace=None  xnstates=0  xfirststate=0  xinitial=0
  Divide : Product  Inputs=*/
  Divide1 : Product  Inputs=*/
  MATLAB Function : MATLAB Function  TreatAsAtomicUnit=on
  Multiply : Product
  Multiply1 : Product
  Read CM Dict : CarMaker4SL/Read CM Dict  xname=Car.muRoadRL  xsync=off
  Read CM Dict1 : CarMaker4SL/Read CM Dict  xname=Car.muRoadRR  xsync=off
  Saturation : Saturate  UpperLimit=10  LowerLimit=-10
  Switch : Switch  Criteria=u2 > Threshold  Threshold=1
  Tunability Factor : Constant
  Write CM Dict : CarMaker4SL/Write CM Dict  xname=maxYawRate  xsync=off
  Write CM Dict1 : CarMaker4SL/Write CM Dict  xname=DesYawRate  xsync=off
  g : Constant  Value=9.81
  Reference Yaw Rate : Outport  VectorParamsAs1DForOutWhenUnconnected=off
  wires:
  Desired Yaw Rate/1 -> Saturation/1
  MATLAB Function/1(ref_yaw) -> Reference Yaw Rate/1  "Reference Yaw Rate"
  Read CM Dict1/1 -> Add/2
  Read CM Dict/1 -> Add/1
  Add/1 -> Divide/1
  Constant/1 -> Divide/2
  Divide/1 -> Multiply/1  "mu (avg)"
  Multiply/1 -> Divide1/1
  Vehicle.v/1 -> Switch/2, Divide1/2
  g/1 -> Multiply/2
  Tunability Factor/1 -> Multiply1/2
  Multiply1/1 -> Write CM Dict/1, MATLAB Function/1(max_yaw)  "Max Yaw Rate"
  Divide1/1 -> Switch/1
  Constant1/1 -> Switch/3
  Switch/1 -> Multiply1/1
  Saturation/1 -> Write CM Dict1/1, MATLAB Function/2(des_yaw)

== system genericjosephtest/CarMaker/IPG Vehicle/PowerTrain/MyPowerTrainXWD/Subsystem ==
  Velocity : Inport  ClipboardFcn=set_param(gcb,'BackgroundColor','red');
  Steering Angle : Inport  Port=2
  Yaw Rate : Inport  Port=3
  Convergence : Scope
  Demux : Demux
  Desired Yaw Rate Generator : Subsystem
  Open-Loop PID Autotuner : slctrlblks/Open-Loop PID Autotuner  PIDType=PIDF  PIDForm=Parallel  TimeDomain=discrete-time  DiscreteTs=0.1  IntegratorFormula=Forward Euler  FilterFormula=Forward Euler  ContinuousTs=0.02  Bandwidth=2  UseExternalWC=off  TargetPM=60  UseExternalPM=off  UseExternalAchievedPM=off  AmpSine=0.1  UseExternalAmpSine=off  EstimateDCGain=on  AmpStep=0.1  UseExternalAmpStep=off  UseExternalFRD=off  UseExternalU0=off  UseExternalDCGain=off  NotDeployTuningModule=off  UsePLCCoder=off  BlockDataType=double  UseConnectedPID=on  blockpath=[]  tunedP=0  tunedI=0  tunedD=0  tunedN=100  tunedPM=0  EstimationWindowSize=4
      settings: SourceProductBaseCode=SD
  "PID Controller " : pid_lib/PID Controller  Controller=PID  Form=Parallel  TimeDomain=Continuous-time  UseExternalTs=off  SampleTime=-1  IntegratorMethod=Forward Euler  FilterMethod=Forward Euler  ControllerParametersSource=external  P=140  I=2312  D=0.85  UseFilter=on  N=47  TunerSelectOption=Transfer Function Based (PID Tuner App)  InitialConditionSource=internal  InitialConditionForIntegrator=0  InitialConditionForFilter=0  DifferentiatorICPrevScaledInput=0  ExternalReset=none  TrackingMode=on  Kt=1  LimitOutput=off  SatLimitsSource=internal  UpperSaturationLimit=240  LowerSaturationLimit=0  LinearizeAsGain=off  AntiWindupMode=clamping  Kb=1  POutMin=[]  POutMax=[]  IOutMin=[]  IOutMax=[]  DOutMin=[]  DOutMax=[]  NOutMin=[]  NOutMax=[]  SumOutMin=[]  SumOutMax=[]  SaturationOutMin=[]  SaturationOutMax=[]  PParamMin=[]  PParamMax=[]  IParamMin=[]  IParamMax=[]  DParamMin=[]  DParamMax=[]  NParamMin=[]  NParamMax=[]  KbParamMin=[]  KbParamMax=[]  KtParamMin=[]  KtParamMax=[]  KbOutMin=[]  KbOutMax=[]  KtOutMin=[]  KtOutMax=[]  IntegratorOutMin=[]  IntegratorOutMax=[]  FilterOutMin=[]  FilterOutMax=[]  SumI1OutMin=[]  SumI1OutMax=[]  SumI2OutMin=[]  SumI2OutMax=[]  SumI3OutMin=[]  SumI3OutMax=[]  SumI4OutMin=[]  SumI4OutMax=[]  SumDOutMin=[]  SumDOutMax=[]  DifferentiatorOutMin=[]  DifferentiatorOutMax=[]  FilterDiffOutCoefMin=[]  FilterDiffOutCoefMax=[]  ReciprocalOutMin=[]  ReciprocalOutMax=[]  SumDenOutMin=[]  SumDenOutMax=[]  SumNumOutMin=[]  SumNumOutMax=[]  DivideOutMin=[]  DivideOutMax=[]  UdiffTsProdOutMin=[]  UdiffTsProdOutMax=[]  NTsProdOutMin=[]  NTsProdOutMax=[]  UintegralTsProdOutMin=[]  UintegralTsProdOutMax=[]  UngainTsProdOutMin=[]  UngainTsProdOutMax=[]  IntegratorContinuousStateAttributes=''  IntegratorStateMustResolveToSignalObject=off  IntegratorRTWStateStorageClass=Auto  FilterContinuousStateAttributes=''  FilterStateMustResolveToSignalObject=off  FilterRTWStateStorageClass=Auto  ParallelPVariant=ExternalParameters  IdealPVariant=Disabled  IVariant=ExternalParameters  DVariant=ExternalParameters  IntegratorVariant=Continuous  SatVariant=Disabled  AWVariant=Passthrough  PCopyVariant=Disabled  TRVariant=Enabled  FdbkBlocksVariant=Forward  IdealPFdbkVariant=Disabled  SatFdbkVariant=Disabled  DerivativeFilterVariant=ContFilter  NVariant=ExternalParameters  NCopyVariant=Disabled  FilterICVariant=InternalICsFilter  IntegratorICVariant=InternalICs  ExternalResetVariant=Disabled  TRSumVariant=TrackingMode  SumFdbkVariant=Disabled  SumVariant=Sum_PID  TsampFilterVariant=InternalTs  TsampNgainVariant=Passthrough  TsampIntegralVariant=Passthrough  ExternalSaturationOutDataTypeStr=Inherit: Same as second input
  PID Gains : Display
      settings: Decimation=5
  PID Gains Data Store Memory : DataStoreMemory  DataStoreName=Gains  InitialValue=[120 120 120 120]  ShowAdditionalParam=off
  Read PID Gains : DataStoreRead  DataStoreName=Gains  DataStoreElements=Gains(:)  IndexOptions=Index vector (dialog)  Indices=1  OutputSizes=1
  Reference Yaw Rate Limiter : Subsystem
  Subtract : Sum  Inputs=+-
  Sum3 : Sum  Inputs=|++
  Update PID Gains : Subsystem
  start tuning1 : Step  Time=10  SampleTime=0
  stop tuning1 : Step  Time=28  After=-1  SampleTime=0
  Trq_R : Outport
  Trq_L : Outport  Port=2
  wires:
  start tuning1/1 -> Sum3/1
  Sum3/1 -> Update PID Gains/Trigger, Open-Loop PID Autotuner/3
  "PID Controller "/1 -> Open-Loop PID Autotuner/1  "Delta Torque command"
  Desired Yaw Rate Generator/1(Desired Yaw Rate) -> Reference Yaw Rate Limiter/2(Desired Yaw Rate)  "Desired Yaw Rate"
  Read PID Gains/1 -> Demux/1, PID Gains/1
  Open-Loop PID Autotuner/1 -> "PID Controller "/6
  Demux/4 -> "PID Controller "/5
  stop tuning1/1 -> Sum3/2
  Subtract/1 -> "PID Controller "/1
  Open-Loop PID Autotuner/3 -> Update PID Gains/1(In1)
  Demux/3 -> "PID Controller "/4
  Yaw Rate/1 -> Open-Loop PID Autotuner/2, Subtract/2  "Yaw Rate Feedback"
  Demux/2 -> "PID Controller "/3
  Open-Loop PID Autotuner/2 -> Convergence/1
  Demux/1 -> "PID Controller "/2
  Velocity/1 -> Desired Yaw Rate Generator/1(Linear Car Velocity), Reference Yaw Rate Limiter/1(Vehicle Velocity)  "Vehicle Velocity"
  Steering Angle/1 -> Desired Yaw Rate Generator/2(steering angle)
  Reference Yaw Rate Limiter/1(Reference Yaw Rate) -> Subtract/1

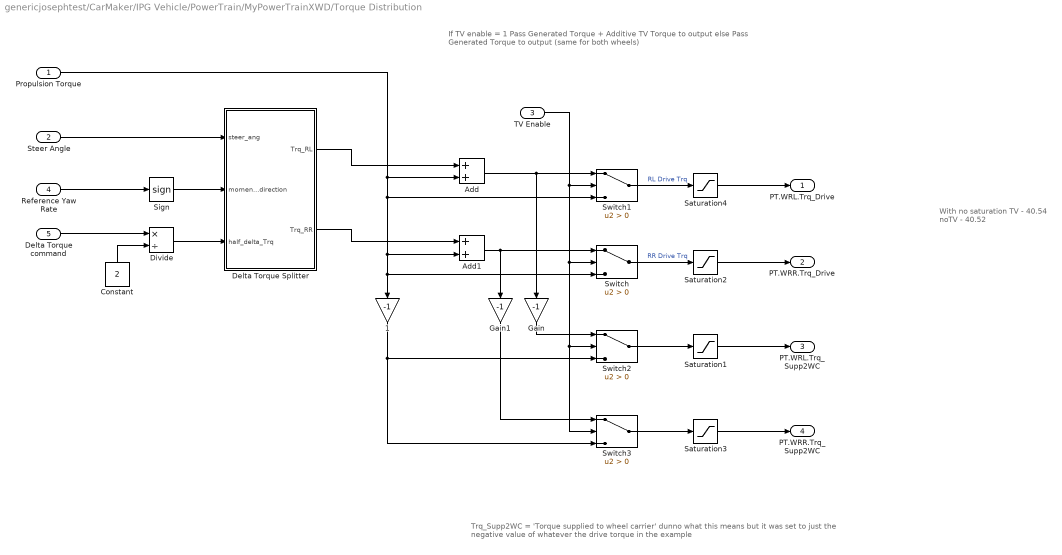
== system genericjosephtest/CarMaker/IPG Vehicle/PowerTrain/MyPowerTrainXWD/Torque Distribution ==
  note: With no saturation
      | TV - 40.54
      | noTV - 40.52
  note: If TV enable = 1
      | Pass Generated Torque + Additive TV Torque to output
      | else
      | Pass Generated Torque to output (same for both wheels)
  note: Trq_Supp2WC = 'Torque supplied to wheel carrier'
      | dunno what this means but it was set to just the negative value of whatever the drive torque in the example
  Propulsion Torque : Inport
  Steer Angle : Inport  Port=2
  TV Enable : Inport  Port=3
  Reference Yaw Rate : Inport  Port=4
  Delta Torque command : Inport  Port=5
  "  1" : Gain  Gain=-1
  Add : Sum
  Add1 : Sum
  Constant : Constant  Value=2
  Delta Torque Splitter : MATLAB Function  TreatAsAtomicUnit=on
  Divide : Product  Inputs=*/
  Gain : Gain  Gain=-1
  Gain1 : Gain  Gain=-1
  Saturation1 : Saturate  UpperLimit=0  LowerLimit=-240
  Saturation2 : Saturate  UpperLimit=240  LowerLimit=0
  Saturation3 : Saturate  UpperLimit=0  LowerLimit=-240
  Saturation4 : Saturate  UpperLimit=240  LowerLimit=0
  Sign : Signum
  Switch{,1..3} (4 alike) : Switch  Criteria=u2 > Threshold
  PT.WRL.Trq_Drive : Outport  VectorParamsAs1DForOutWhenUnconnected=off
  PT.WRR.Trq_Drive : Outport  Port=2  VectorParamsAs1DForOutWhenUnconnected=off
  PT.WRL.Trq_Supp2WC : Outport  Port=3  VectorParamsAs1DForOutWhenUnconnected=off
  PT.WRR.Trq_Supp2WC : Outport  Port=4  VectorParamsAs1DForOutWhenUnconnected=off
  wires:
  Gain1/1 -> Switch3/1
  "  1"/1 -> Switch2/3, Switch3/3
  Add/1 -> Switch1/1, Gain/1
  Divide/1 -> Delta Torque Splitter/3(half_delta_Trq)
  Propulsion Torque/1 -> Switch1/3, "  1"/1, Switch/3, Add1/2, Add/2
  TV Enable/1 -> Switch1/2, Switch/2, Switch3/2, Switch2/2
  Delta Torque command/1 -> Divide/1
  Delta Torque Splitter/1(Trq_RL) -> Add/1
  Add1/1 -> Switch/1, Gain1/1
  Sign/1 -> Delta Torque Splitter/2(moment_direction)
  Constant/1 -> Divide/2
  Delta Torque Splitter/2(Trq_RR) -> Add1/1
  Gain/1 -> Switch2/1
  Reference Yaw Rate/1 -> Sign/1
  Switch3/1 -> Saturation3/1
  Saturation3/1 -> PT.WRR.Trq_Supp2WC/1
  Switch1/1 -> Saturation4/1  "RL Drive Trq"
  Switch/1 -> Saturation2/1  "RR Drive Trq"
  Switch2/1 -> Saturation1/1
  Saturation1/1 -> PT.WRL.Trq_Supp2WC/1
  Saturation4/1 -> PT.WRL.Trq_Drive/1
  Saturation2/1 -> PT.WRR.Trq_Drive/1
  Steer Angle/1 -> Delta Torque Splitter/1(steer_ang)

== system genericjosephtest/CarMaker/IPG Vehicle/PowerTrain/MyPowerTrainXWD/Update PID Gains ==
  In1 : Inport
  Trigger : TriggerPort  TriggerType=falling  VariantControl=Variant  PortDimensions=1
  Bus Selector : BusSelector  OutputSignals=P,I,D,N
  Mux : Mux
  Write PID Gains : DataStoreWrite  DataStoreName=Gains  DataStoreElements=Gains(:)  IndexOptions=Index vector (dialog)  Indices=1  OutputSizes=1
  wires:
  Mux/1 -> Write PID Gains/1
  Bus Selector/2 -> Mux/2  "<I>"
  Bus Selector/1 -> Mux/1  "<P>"
  In1/1 -> Bus Selector/1
  Bus Selector/3 -> Mux/3  "<D>"
  Bus Selector/4 -> Mux/4  "<N>"

== system genericjosephtest/CarMaker/IPG Vehicle/PowerTrain/MyPowerTrainXWD/ts_18 Gain Scheduler (PIDN Lookup) ==
  Vhcl.v : Inport
  Kd Lookup : Lookup_n-D  NumberOfTableDimensions=1  BreakpointsForDimension1=[1,3,5,7,9,11,13,15]  Table=[0,0,0,0,0,-0.40505,-0.50277,-1.0544]  InternalRulePriority=Speed  RndMeth=Simplest  InputSameDT=on
  Ki Lookup : Lookup_n-D  NumberOfTableDimensions=1  BreakpointsForDimension1=[1,3,5,7,9,11,13,15]  Table=[37865.65,10454.7184,5331.6587,8450.1199,7889.3391,7361.3561,6813.2147,6310.914]  InternalRulePriority=Speed  RndMeth=Simplest  InputSameDT=on
  Kp Lookup : Lookup_n-D  NumberOfTableDimensions=1  BreakpointsForDimension1=[1,3,5,7,9,11,13,15]  Table=[0,0,0,127.0119,171.5424,208.4617,225.764,251.3245]  InternalRulePriority=Speed  RndMeth=Simplest  InputSameDT=on
  Mux : Mux
  N Lookup : Lookup_n-D  NumberOfTableDimensions=1  BreakpointsForDimension1=[1,3,5,7,9,11,13,15]  Table=[0,0,0,0,0,31.6952,27.1972,27.1927]  InternalRulePriority=Speed  RndMeth=Simplest  InputSameDT=on
  PIDN Gains : Outport  VectorParamsAs1DForOutWhenUnconnected=off
  wires:
  Kd Lookup/1 -> Mux/3
  Vhcl.v/1 -> N Lookup/1, Kd Lookup/1, Kp Lookup/1, Ki Lookup/1
  Ki Lookup/1 -> Mux/2
  Kp Lookup/1 -> Mux/1
  N Lookup/1 -> Mux/4
  Mux/1 -> PIDN Gains/1

== system genericjosephtest/CarMaker/IPG Vehicle/PowerTrain/MyPowerTrainXWD/ts_18 Gain Scheduler (PIDN Lookup) v2 19sep ==
  Vhcl.v : Inport
  Kd Lookup : Lookup_n-D  NumberOfTableDimensions=1  BreakpointsForDimension1=[1,3,5,7,9,11,13,15]  Table=[0,0,0,0,0,-1.854,-1.907,-0.07946]  InternalRulePriority=Speed  RndMeth=Simplest  InputSameDT=on
  Ki Lookup : Lookup_n-D  NumberOfTableDimensions=1  BreakpointsForDimension1=[1,3,5,7,9,11,13,15]  Table=[67967.36,20046.34,10353.28,11261.09,10979.136,9397.25,9272.36,11112.25]  InternalRulePriority=Speed  RndMeth=Simplest  InputSameDT=on
  Kp Lookup : Lookup_n-D  NumberOfTableDimensions=1  BreakpointsForDimension1=[1,3,5,7,9,11,13,15]  Table=[0,0,0,49.142,124.61,186.37,233.8,316.28]  InternalRulePriority=Speed  RndMeth=Simplest  InputSameDT=on
  Mux : Mux
  N Lookup : Lookup_n-D  NumberOfTableDimensions=1  BreakpointsForDimension1=[1,3,5,7,9,11,13,15]  Table=[100,100,100,100,100,25.58,33.73,3980.08]  InternalRulePriority=Speed  RndMeth=Simplest  InputSameDT=on
  PIDN Gains : Outport  VectorParamsAs1DForOutWhenUnconnected=off
  wires:
  Kd Lookup/1 -> Mux/3
  Vhcl.v/1 -> N Lookup/1, Kd Lookup/1, Kp Lookup/1, Ki Lookup/1
  Ki Lookup/1 -> Mux/2
  Kp Lookup/1 -> Mux/1
  N Lookup/1 -> Mux/4
  Mux/1 -> PIDN Gains/1

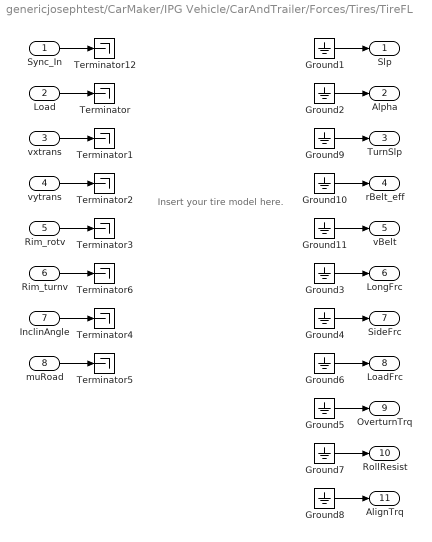
== system genericjosephtest/CarMaker/IPG Vehicle/CarAndTrailer/Forces/Tires/TireFL ==
  note: Insert your tire model here.
  Sync_In : Inport
  Load : Inport  Port=2
  vxtrans : Inport  Port=3
  vytrans : Inport  Port=4
  Rim_rotv : Inport  Port=5
  Rim_turnv : Inport  Port=6
  InclinAngle : Inport  Port=7
  muRoad : Inport  Port=8
  Ground{1..11} (11 alike) : Ground
  Terminator{,1..6,12} (8 alike) : Terminator
  Slp : Outport  VectorParamsAs1DForOutWhenUnconnected=off
  Alpha : Outport  Port=2  VectorParamsAs1DForOutWhenUnconnected=off
  TurnSlp : Outport  Port=3  VectorParamsAs1DForOutWhenUnconnected=off
  rBelt_eff : Outport  Port=4  VectorParamsAs1DForOutWhenUnconnected=off
  vBelt : Outport  Port=5  VectorParamsAs1DForOutWhenUnconnected=off
  LongFrc : Outport  Port=6  VectorParamsAs1DForOutWhenUnconnected=off
  SideFrc : Outport  Port=7  VectorParamsAs1DForOutWhenUnconnected=off
  LoadFrc : Outport  Port=8  VectorParamsAs1DForOutWhenUnconnected=off
  OverturnTrq : Outport  Port=9  VectorParamsAs1DForOutWhenUnconnected=off
  RollResist : Outport  Port=10  VectorParamsAs1DForOutWhenUnconnected=off
  AlignTrq : Outport  Port=11  VectorParamsAs1DForOutWhenUnconnected=off
  wires:
  Ground11/1 -> vBelt/1
  Ground10/1 -> rBelt_eff/1
  Ground9/1 -> TurnSlp/1
  Rim_turnv/1 -> Terminator6/1
  Sync_In/1 -> Terminator12/1
  Ground2/1 -> Alpha/1
  Ground3/1 -> LongFrc/1
  Ground4/1 -> SideFrc/1
  Ground5/1 -> OverturnTrq/1
  vxtrans/1 -> Terminator1/1
  vytrans/1 -> Terminator2/1
  Rim_rotv/1 -> Terminator3/1
  InclinAngle/1 -> Terminator4/1
  muRoad/1 -> Terminator5/1
  Load/1 -> Terminator/1
  Ground1/1 -> Slp/1
  Ground6/1 -> LoadFrc/1
  Ground7/1 -> RollResist/1
  Ground8/1 -> AlignTrq/1

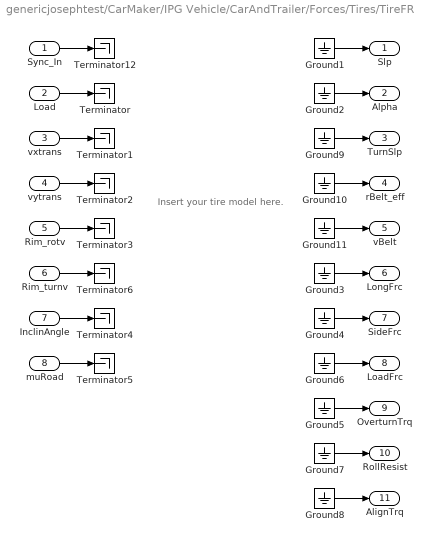
== system genericjosephtest/CarMaker/IPG Vehicle/CarAndTrailer/Forces/Tires/TireFR ==
  note: Insert your tire model here.
  Sync_In : Inport
  Load : Inport  Port=2
  vxtrans : Inport  Port=3
  vytrans : Inport  Port=4
  Rim_rotv : Inport  Port=5
  Rim_turnv : Inport  Port=6
  InclinAngle : Inport  Port=7
  muRoad : Inport  Port=8
  Ground{1..11} (11 alike) : Ground
  Terminator{,1..6,12} (8 alike) : Terminator
  Slp : Outport  VectorParamsAs1DForOutWhenUnconnected=off
  Alpha : Outport  Port=2  VectorParamsAs1DForOutWhenUnconnected=off
  TurnSlp : Outport  Port=3  VectorParamsAs1DForOutWhenUnconnected=off
  rBelt_eff : Outport  Port=4  VectorParamsAs1DForOutWhenUnconnected=off
  vBelt : Outport  Port=5  VectorParamsAs1DForOutWhenUnconnected=off
  LongFrc : Outport  Port=6  VectorParamsAs1DForOutWhenUnconnected=off
  SideFrc : Outport  Port=7  VectorParamsAs1DForOutWhenUnconnected=off
  LoadFrc : Outport  Port=8  VectorParamsAs1DForOutWhenUnconnected=off
  OverturnTrq : Outport  Port=9  VectorParamsAs1DForOutWhenUnconnected=off
  RollResist : Outport  Port=10  VectorParamsAs1DForOutWhenUnconnected=off
  AlignTrq : Outport  Port=11  VectorParamsAs1DForOutWhenUnconnected=off
  wires:
  Ground11/1 -> vBelt/1
  Ground10/1 -> rBelt_eff/1
  Ground9/1 -> TurnSlp/1
  Rim_turnv/1 -> Terminator6/1
  Sync_In/1 -> Terminator12/1
  Ground2/1 -> Alpha/1
  Ground3/1 -> LongFrc/1
  Ground4/1 -> SideFrc/1
  Ground5/1 -> OverturnTrq/1
  vxtrans/1 -> Terminator1/1
  vytrans/1 -> Terminator2/1
  Rim_rotv/1 -> Terminator3/1
  InclinAngle/1 -> Terminator4/1
  muRoad/1 -> Terminator5/1
  Load/1 -> Terminator/1
  Ground1/1 -> Slp/1
  Ground6/1 -> LoadFrc/1
  Ground7/1 -> RollResist/1
  Ground8/1 -> AlignTrq/1
